simulink model "general_bristle_model_2d"  (R2021b)
settings: Solver=VariableStepAuto  StartTime=0.0  StopTime=t_end  FixedStep=t_step  MaxStep=t_step  RelTol=1e-3  AbsTol=1e-3
libraries: nesl_utility x2
settings Model: Creator=Q657093  LastModifiedBy=Q657093
settings SolverCC: AutoScaleAbsTol=off  ZeroCrossAlgorithm=Adaptive  AlgebraicLoopSolver=TrustRegion
settings DataIOCC: SaveFinalState=on  SaveState=on  InspectSignalLogs=on
settings DebuggingCC: IgnoredZcDiagnostic=none  SymbolicDimsDataTypeCodeGenerationDiagnostic=none
settings SFSimCC: CustomCodeUndefinedFunction=UseInterfaceOnly
settings SimscapeCC: ExplicitSolverDiagnosticOptions=none  SimscapeLogType=all  SimscapeLogSimulationStatistics=on  SimscapeLogToSDI=on  SimscapeLogLimitData=off  SimscapeLogDataHistory=10000

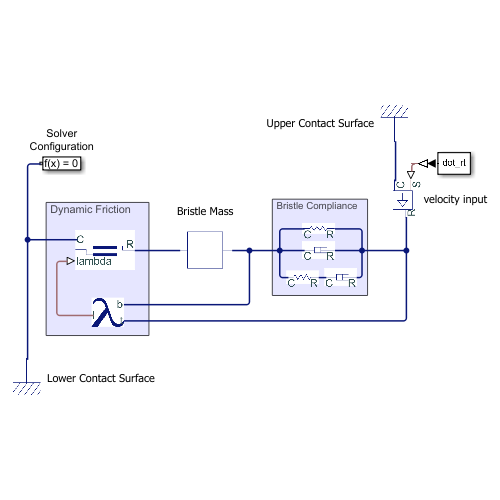
[thumbnail: Simulink's stored preview of the top-level diagram]
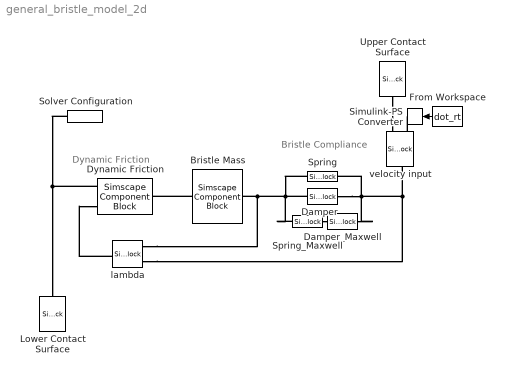
== system general_bristle_model_2d ==
  note: Bristle Compliance
  note: Dynamic Friction
  Bristle Mass : SimscapeComponentBlock  SourceFile=mass2d  ComponentPath=mass2d  ComponentVariants="[\"mass2d\"]"  ComponentVariantNames="[\"mass2d\"]"  ClassName=mass2d  SchemaVersion=1  mass=m_b kg  num_ports=foundation.enum.numPorts2.two  v_specify=off  v_priority=High  v=[0, 0] m/s  v_nominal_specify=off  v_nominal_unit=m/s  v_nominal_value=1  f_specify=off  f_priority=None  f=[0, 0] N  f_nominal_specify=off  f_nominal_unit=N  f_nominal_value=1
      settings: CopyFcn=simscape.engine.sli.internal.componentblockcallback(gcbh,'COPY')  PreCopyFcn=simscape.engine.sli.internal.componentblockcallback(gcbh,'PRECOPY')  PreDeleteFcn=simscape.engine.sli.internal.componentblockcallback(gcbh,'PREDELETE')  InternalSimscapePortConfiguration="{\"Bottom\":[],\"Left\":[{\"id\":\"M\",\"label\":\"\",\"type\":\"translational2d\"}],\"Right\":[{\"id\":\"N\",\"label\":\"\",\"type\":\"translational2d\"}],\"Top\":[]}"
      mask Type: Mass
  Damper : SimscapeComponentBlock  SourceFile=damper2d  ComponentPath=damper2d  ComponentVariants="[\"damper2d\"]"  ComponentVariantNames="[\"damper2d\"]"  ClassName=damper2d  SchemaVersion=1  dmp_rate=d N/(m/s)  v_specify=off  v_priority=None  v=[0; 0] m/s  v_nominal_specify=off  v_nominal_unit=m/s  v_nominal_value=1  f_specify=off  f_priority=None  f=[0; 0] N  f_nominal_specify=off  f_nominal_unit=N  f_nominal_value=1  x_specify=off  x_priority=High  x=[0; 0] m  x_nominal_specify=off  x_nominal_unit=m  x_nominal_value=1
      settings: CopyFcn=simscape.engine.sli.internal.componentblockcallback(gcbh,'COPY')  PreCopyFcn=simscape.engine.sli.internal.componentblockcallback(gcbh,'PRECOPY')  PreDeleteFcn=simscape.engine.sli.internal.componentblockcallback(gcbh,'PREDELETE')  InternalSimscapePortConfiguration="{\"Bottom\":[],\"Left\":[{\"id\":\"R\",\"label\":\"R\",\"type\":\"translational2d\"}],\"Right\":[{\"id\":\"C\",\"label\":\"C\",\"type\":\"translational2d\"}],\"Top\":[]}"
      mask Type: damper2d
  Damper_Maxwell : SimscapeComponentBlock  SourceFile=damper2d  ComponentPath=damper2d  ComponentVariants="[\"damper2d\"]"  ComponentVariantNames="[\"damper2d\"]"  ClassName=damper2d  SchemaVersion=1  dmp_rate=d_m N/(m/s)  v_specify=off  v_priority=None  v=[0; 0] m/s  v_nominal_specify=off  v_nominal_unit=m/s  v_nominal_value=1  f_specify=off  f_priority=None  f=[0; 0] N  f_nominal_specify=off  f_nominal_unit=N  f_nominal_value=1  x_specify=off  x_priority=High  x=[0; 0] m  x_nominal_specify=off  x_nominal_unit=m  x_nominal_value=1
      settings: CopyFcn=simscape.engine.sli.internal.componentblockcallback(gcbh,'COPY')  PreCopyFcn=simscape.engine.sli.internal.componentblockcallback(gcbh,'PRECOPY')  PreDeleteFcn=simscape.engine.sli.internal.componentblockcallback(gcbh,'PREDELETE')  InternalSimscapePortConfiguration="{\"Bottom\":[],\"Left\":[{\"id\":\"R\",\"label\":\"R\",\"type\":\"translational2d\"}],\"Right\":[{\"id\":\"C\",\"label\":\"C\",\"type\":\"translational2d\"}],\"Top\":[]}"
      mask Type: damper2d
  Dynamic Friction : SimscapeComponentBlock  SourceFile=dynamic_friction2d  ComponentPath=dynamic_friction2d  ComponentVariants="[\"dynamic_friction2d\"]"  ComponentVariantNames="[\"dynamic_friction2d\"]"  ClassName=dynamic_friction2d  SchemaVersion=1  F_g=F_g N  F_h=F_h N  v_minslip=v_minslip m/s  lambda_flag=lambda_flag  v_specify=off  v_priority=None  v=[0; 0] m/s  v_nominal_specify=off  v_nominal_unit=m/s  v_nominal_value=1  f_specify=off  f_priority=None  f=[0; 0] N  f_nominal_specify=off  f_nominal_unit=N  f_nominal_value=1  stick_specify=on  stick_priority=None  stick=1
      settings: CopyFcn=simscape.engine.sli.internal.componentblockcallback(gcbh,'COPY')  PreCopyFcn=simscape.engine.sli.internal.componentblockcallback(gcbh,'PRECOPY')  PreDeleteFcn=simscape.engine.sli.internal.componentblockcallback(gcbh,'PREDELETE')  InternalSimscapePortConfiguration="{\"Bottom\":[],\"Left\":[{\"id\":\"R\",\"label\":\"R\",\"type\":\"translational2d\"}],\"Right\":[{\"id\":\"C\",\"label\":\"C\",\"type\":\"translational2d\"},{\"id\":\"lambda\",\"label\":\"lambda\",\"type\":\"input\"}],\"Top\":[]}"
      mask Type: Translational Friction
  From Workspace : FromWorkspace  VariableName=dot_rt  SampleTime=-1  OutputAfterFinalValue=Holding final value
  Lower Contact Surface : SimscapeComponentBlock  SourceFile=reference2d  ComponentPath=reference2d  ComponentVariants="[\"reference2d\"]"  ComponentVariantNames="[\"reference2d\"]"  ClassName=reference2d  SchemaVersion=1
      settings: CopyFcn=simscape.engine.sli.internal.componentblockcallback(gcbh,'COPY')  PreCopyFcn=simscape.engine.sli.internal.componentblockcallback(gcbh,'PRECOPY')  PreDeleteFcn=simscape.engine.sli.internal.componentblockcallback(gcbh,'PREDELETE')  InternalSimscapePortConfiguration="{\"Bottom\":[],\"Left\":[{\"id\":\"V\",\"label\":\"\",\"type\":\"translational2d\"}],\"Right\":[],\"Top\":[]}"
      mask Type: Mechanical Translational Reference
  Simulink-PS Converter : nesl_utility/Simulink-PS Converter  PhysicalDomain=network_engine_domain  SubClassName=ps_input  LeftPortType=input  RightPortType=output  PseudoPeriodic=off  Frequencies=[]  NoiseDistribution=none  NoiseParameters=[]  Unit=1  AffineConversion=off  FilteringAndDerivatives=provide  SimscapeFilterOrder=1  InputFilterTimeConstant=0.001  UdotUserProvided=0
      settings: SourceProductBaseCode=PW,SS
  Solver Configuration : nesl_utility/Solver Configuration  PhysicalDomain=network_engine_domain  SubClassName=solver  LeftPortType=input  RightPortType=generic  Tones=[]  Harmonics=[]  SimulateNoise=off  Profile=off  UseLocalSampling=off  EnableSwitchedLinearOptims=on  FrequencyDomain=off  UseCCode=off  RelTol=0.001  AbsTol=1e-06  MinStep=1e-09  ToWorkspace=off  RevertToSquareIcSolve=off  NumHomotopyIterations=100  PhasorMode=off  PhasorModeNumHarmonics=1  DoDC=off  ResidualTolerance=1e-09  UseLocalSolver=on  LocalSolverChoice=NE_BACKWARD_EULER_ADVANCER  LocalSolverSampleTime=t_step  DoFixedCost=on  MaxNonlinIter=3  MaxModeIter=2  ComputeImpulses=off  ImpulseIterations=2  LinearAlgebra=auto  EquationFormulation=NE_TIME_EF  DelaysMemoryBudget=1024  AutomaticFiltering=on  FilteringTimeConstant=t_step  PartitionStorageMethod=AS_NEEDED  PartitionMemoryBudget=1024  PartitionMethod=ROBUST
      settings: SourceProductBaseCode=PW,SS
  Spring : SimscapeComponentBlock  SourceFile=spring2d  ComponentPath=spring2d  ComponentVariants="[\"spring2d\"]"  ComponentVariantNames="[\"spring2d\"]"  ClassName=spring2d  SchemaVersion=1  spr_rate=k N/m  v_specify=off  v_priority=None  v=[0, 0] m/s  v_nominal_specify=off  v_nominal_unit=m/s  v_nominal_value=1  f_specify=off  f_priority=None  f=[0, 0] N  f_nominal_specify=off  f_nominal_unit=N  f_nominal_value=1  x_specify=off  x_priority=High  x=0 m  x_nominal_specify=off  x_nominal_unit=m  x_nominal_value=1
      settings: CopyFcn=simscape.engine.sli.internal.componentblockcallback(gcbh,'COPY')  PreCopyFcn=simscape.engine.sli.internal.componentblockcallback(gcbh,'PRECOPY')  PreDeleteFcn=simscape.engine.sli.internal.componentblockcallback(gcbh,'PREDELETE')  InternalSimscapePortConfiguration="{\"Bottom\":[],\"Left\":[{\"id\":\"R\",\"label\":\"R\",\"type\":\"translational2d\"}],\"Right\":[{\"id\":\"C\",\"label\":\"C\",\"type\":\"translational2d\"}],\"Top\":[]}"
      mask Type: Translational Spring
  Spring_Maxwell : SimscapeComponentBlock  SourceFile=spring2d  ComponentPath=spring2d  ComponentVariants="[\"spring2d\"]"  ComponentVariantNames="[\"spring2d\"]"  ClassName=spring2d  SchemaVersion=1  spr_rate=k_m N/m  v_specify=off  v_priority=None  v=[0, 0] m/s  v_nominal_specify=off  v_nominal_unit=m/s  v_nominal_value=1  f_specify=off  f_priority=None  f=[0, 0] N  f_nominal_specify=off  f_nominal_unit=N  f_nominal_value=1  x_specify=off  x_priority=High  x=0 m  x_nominal_specify=off  x_nominal_unit=m  x_nominal_value=1
      settings: CopyFcn=simscape.engine.sli.internal.componentblockcallback(gcbh,'COPY')  PreCopyFcn=simscape.engine.sli.internal.componentblockcallback(gcbh,'PRECOPY')  PreDeleteFcn=simscape.engine.sli.internal.componentblockcallback(gcbh,'PREDELETE')  InternalSimscapePortConfiguration="{\"Bottom\":[],\"Left\":[{\"id\":\"R\",\"label\":\"R\",\"type\":\"translational2d\"}],\"Right\":[{\"id\":\"C\",\"label\":\"C\",\"type\":\"translational2d\"}],\"Top\":[]}"
      mask Type: Translational Spring
  Upper Contact Surface : SimscapeComponentBlock  SourceFile=reference2d  ComponentPath=reference2d  ComponentVariants="[\"reference2d\"]"  ComponentVariantNames="[\"reference2d\"]"  ClassName=reference2d  SchemaVersion=1
      settings: CopyFcn=simscape.engine.sli.internal.componentblockcallback(gcbh,'COPY')  PreCopyFcn=simscape.engine.sli.internal.componentblockcallback(gcbh,'PRECOPY')  PreDeleteFcn=simscape.engine.sli.internal.componentblockcallback(gcbh,'PREDELETE')  InternalSimscapePortConfiguration="{\"Bottom\":[],\"Left\":[{\"id\":\"V\",\"label\":\"\",\"type\":\"translational2d\"}],\"Right\":[],\"Top\":[]}"
      mask Type: Mechanical Translational Reference
  lambda : SimscapeComponentBlock  SourceFile=lambda2d  ComponentPath=lambda2d  ComponentVariants="[\"lambda2d\"]"  ComponentVariantNames="[\"lambda2d\"]"  ClassName=lambda2d  SchemaVersion=1  F_g=F_g N  lambda_flag=lambda_flag
      settings: CopyFcn=simscape.engine.sli.internal.componentblockcallback(gcbh,'COPY')  PreCopyFcn=simscape.engine.sli.internal.componentblockcallback(gcbh,'PRECOPY')  PreDeleteFcn=simscape.engine.sli.internal.componentblockcallback(gcbh,'PREDELETE')  InternalSimscapePortConfiguration="{\"Bottom\":[],\"Left\":[{\"id\":\"top\",\"label\":\"t\",\"type\":\"translational2d\"},{\"id\":\"bottom\",\"label\":\"b\",\"type\":\"translational2d\"}],\"Right\":[{\"id\":\"l\",\"label\":\"l\",\"type\":\"output\"}],\"Top\":[]}"
      mask Type: lambda
  velocity input : SimscapeComponentBlock  SourceFile=velocity2d  ComponentPath=velocity2d  ComponentVariants="[\"velocity2d\"]"  ComponentVariantNames="[\"velocity2d\"]"  ClassName=velocity2d  SchemaVersion=1
      settings: CopyFcn=simscape.engine.sli.internal.componentblockcallback(gcbh,'COPY')  PreCopyFcn=simscape.engine.sli.internal.componentblockcallback(gcbh,'PRECOPY')  PreDeleteFcn=simscape.engine.sli.internal.componentblockcallback(gcbh,'PREDELETE')  InternalSimscapePortConfiguration="{\"Bottom\":[],\"Left\":[{\"id\":\"R\",\"label\":\"R\",\"type\":\"translational2d\"}],\"Right\":[{\"id\":\"S\",\"label\":\"S\",\"type\":\"input\"},{\"id\":\"C\",\"label\":\"C\",\"type\":\"translational2d\"}],\"Top\":[]}"
      mask Type: Ideal Translational Velocity Source
  wires:
  From Workspace/1 -> Simulink-PS Converter/1
  connections:
  velocity input/RConn1 -- Simulink-PS Converter/RConn1
  lambda/RConn1 -- Dynamic Friction/RConn2
  Dynamic Friction/RConn1 -- Solver Configuration/RConn1 -- Lower Contact Surface/LConn1
  lambda/LConn1 -- velocity input/LConn1 -- Damper_Maxwell/LConn1 -- Spring/LConn1 -- Damper/LConn1
  Spring/RConn1 -- lambda/LConn2 -- Bristle Mass/LConn1 -- Spring_Maxwell/RConn1 -- Damper/RConn1
  Bristle Mass/RConn1 -- Dynamic Friction/LConn1
  Upper Contact Surface/LConn1 -- velocity input/RConn2
  Spring_Maxwell/LConn1 -- Damper_Maxwell/RConn1
